simulink model "control_vectorial_bldc"  (R2024b)
settings: Solver=ode14x  StartTime=0.0  StopTime=1  FixedStep=1e-6  MaxStep=1e-5  MinStep=1e-7  RelTol=1e-4  EnableMultiTasking=on
InitFcn:
  | wksp = get_param('control_vectorial_bldc', 'ModelWorkspace');
  | ref_speed = getVariable(wksp, 'w');
  | pw = getVariable(wksp, 'P_speed');
  | iw = getVariable(wksp, 'I_speed');
  | pq = getVariable(wksp, 'P_torque');
  | pd = getVariable(wksp, 'P_flux');
  | pwm_freq = getVariable(wksp, 'pwm_freq');
  | 
  | y = zeros(4, 1000);
  | 
  | command = strcat('sed -i "s/ref_speed =.*/ref_speed = ',num2str(ref_speed),';/" /home/radu/workspace/no-OS/projects/PID_app/src/examples/ext_loop/ext_loop_example.c');
  | [status,cmdout] = system(command);
  | 
  | command = strcat('sed -i "s/pwm_freq =.*/pwm_freq = ',num2str(pwm_freq),';/" /home/radu/workspace/no-OS/projects/PID_app/src/examples/ext_loop/ext_loop_example.c');
  | [status,cmdout] = system(command);
  | 
  | command = strcat('sed -i "s/kp_speed =.*/kp_speed = ',num2str(pw),';/" /home/radu/workspace/no-OS/projects/PID_app/src/examples/ext_loop/ext_loop_example.c');
  | [status,cmdout] = system(command);
  | 
  | command = strcat('sed -i "s/ki_speed =.*/ki_speed = ',num2str(iw),';/" /home/radu/workspace/no-OS/projects/PID_app/src/examples/ext_loop/ext_loop_example.c');
  | [status,cmdout] = system(command);
  | 
  | command = strcat('sed -i "s/kp_torque =.*/kp_torque = ',num2str(pq),';/" /home/radu/workspace/licenta/SOFTWARE/no-OS/projects/PID_app/src/examples/ext_loop/ext_loop_example.c');
  | [status,cmdout] = system(command);
  | 
  | command = strcat('sed -i "s/kp_flux =.*/kp_flux = ',num2str(pd),';/" /home/radu/workspace/no-OS/projects/PID_app/src/examples/ext_loop/ext_loop_example.c');
  | [status,cmdout] = system(command);
  | 
  | cd '/home/radu/workspace/no-OS/projects/PID_app';
  | 
  | command = 'stty -F /dev/ttyACM0 1000000';
  | [status, cmdout] = system(command);
  | command = 'cat /dev/ttyACM0 > speed_plot.txt & make PLATFORM=stm32 run';
  | [status, cmdout] = system(command);
  | 
  | pause(10);
  | 
  | command = 'pkill -f "cat /dev/ttyACM0"';
  | [status, cmdout] = system(command);
  | 
  | fid = fopen('speed_plot.txt','rt');
  | C = textscan(fid, '%f%f%f%f%f%f%f');
  | fclose(fid);
  | y=cell2mat(C);
  | 
  | ms = table2timetable(table(milliseconds(y(:,1:1)), y(:,2:2)));
  | mt = table2timetable(table(milliseconds(y(:,1:1)), y(:,3:3).*0.000009077));
  | mf = table2timetable(table(milliseconds(y(:,1:1)), y(:,4:4).*0.000009077));
  | ms.Properties.VariableNames{1} = 'Motor Speed';
  | mt.Properties.VariableNames{1} = 'Motor Torque';
  | mf.Properties.VariableNames{1} = 'Motor Flux';
  | 
  | command = 'rm speed_plot.txt';
  | [status, cmdout] = system(command);
model workspace (MAT data in the model file):
  I_speed = 0.006
  P_flux = 0.72
  P_speed = 1.04
  P_torque = 0.72
  pwm_freq = 50000
  w = 2000
libraries: ee_lib x15, nesl_utility x10, fl_lib x5, eeTransforms x3, slpidlib x3, spsSVPWMGenerator2LevelLib x1
(part 2 of 2)

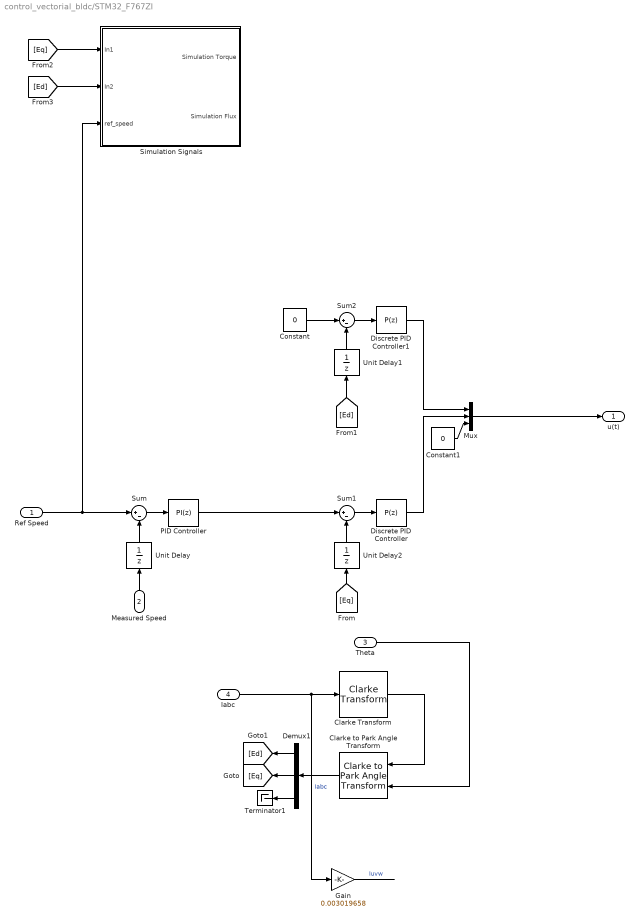
== system control_vectorial_bldc/STM32_F767ZI ==
  Ref Speed : Inport
  Measured Speed : Inport  Port=2
  Theta : Inport  Port=3
  Iabc : Inport  Port=4
  Clarke Transform : eeTransforms/Clarke Transform  PowerInvariant=off
      settings: LibrarySourceBlock=|
      | ee_sl_lib/Mathematical
      | Transforms/Clarke Transform
  Clarke to Park Angle Transform : eeTransforms/Clarke to Park Angle Transform  AxisAlignment=Q-axis
      settings: LibrarySourceBlock=|
      | ee_sl_lib/Mathematical
      | Transforms/Clarke to Park
      | Angle Transform
  Constant : Constant  Value=0
  Constant1 : Constant  Value=0
  Demux1 : Demux  Outputs=3
  Discrete PID Controller : slpidlib/PID Controller  Controller=P  Form=Parallel  TimeDomain=Discrete-time  UseExternalTs=off  SampleTime=-1  IntegratorMethod=Backward Euler  FilterMethod=Forward Euler  ControllerParametersSource=internal  P=P_torque  I=0  UseKiTs=off  D=0  UseExternalDerivativeSource=off  N=100  UseFilter=on  TunerSelectOption=Transfer Function Based (PID Tuner App)  InitialConditionSource=internal  InitialConditionForIntegrator=0  InitialConditionForFilter=0  DifferentiatorICPrevScaledInput=0  ExternalReset=none  TrackingMode=off  Kt=1  LimitOutput=off  SatLimitsSource=internal  UpperSaturationLimit=inf  LowerSaturationLimit=-inf  LinearizeAsGain=off  AntiWindupMode=none  Kb=1  LimitIntegrator=off  UpperIntegratorSaturationLimit=inf  LowerIntegratorSaturationLimit=-inf  POutMin=[]  POutMax=[]  IOutMin=[]  IOutMax=[]  DOutMin=[]  DOutMax=[]  NOutMin=[]  NOutMax=[]  SumOutMin=[]  SumOutMax=[]  SaturationOutMin=[]  SaturationOutMax=[]  PParamMin=[]  PParamMax=[]  IParamMin=[]  IParamMax=[]  DParamMin=[]  DParamMax=[]  NParamMin=[]  NParamMax=[]  KbParamMin=[]  KbParamMax=[]  KtParamMin=[]  KtParamMax=[]  KbOutMin=[]  KbOutMax=[]  KtOutMin=[]  KtOutMax=[]  IntegratorOutMin=[]  IntegratorOutMax=[]  FilterOutMin=[]  FilterOutMax=[]  SumI1OutMin=[]  SumI1OutMax=[]  SumI2OutMin=[]  SumI2OutMax=[]  SumI3OutMin=[]  SumI3OutMax=[]  SumI4OutMin=[]  SumI4OutMax=[]  SumDOutMin=[]  SumDOutMax=[]  DifferentiatorOutMin=[]  DifferentiatorOutMax=[]  FilterDiffOutCoefMin=[]  FilterDiffOutCoefMax=[]  ReciprocalOutMin=[]  ReciprocalOutMax=[]  SumDenOutMin=[]  SumDenOutMax=[]  SumNumOutMin=[]  SumNumOutMax=[]  DivideOutMin=[]  DivideOutMax=[]  UdiffTsProdOutMin=[]  UdiffTsProdOutMax=[]  NTsProdOutMin=[]  NTsProdOutMax=[]  UintegralTsProdOutMin=[]  UintegralTsProdOutMax=[]  UngainTsProdOutMin=[]  UngainTsProdOutMax=[]  ClampingZeroOutDataTypeStr=Inherit: Inherit via back propagation  ClampingZeroOutMin=[]  ClampingZeroOutMax=[]  FilterDenConstantOutDataTypeStr=Inherit: Inherit via back propagation  FilterDenConstantOutMin=[]  FilterDenConstantOutMax=[]  PCopyOutDataTypeStr=Inherit: Inherit via back propagation  PCopyOutMin=[]  PCopyOutMax=[]  NCopyOutDataTypeStr=Inherit: Inherit via back propagation  NCopyOutMin=[]  NCopyOutMax=[]  IntegratorContinuousStateAttributes=''  IntegratorStateMustResolveToSignalObject=off  IntegratorRTWStateStorageClass=Auto  FilterContinuousStateAttributes=''  FilterStateMustResolveToSignalObject=off  FilterRTWStateStorageClass=Auto  ParallelPVariant=InternalParameters  IdealPVariant=Disabled  IVariant=Disabled  DVariant=Disabled  IntegratorVariant=Disabled  SatVariant=Disabled  AWVariant=Disabled  PCopyVariant=Disabled  TRVariant=Disabled  FdbkBlocksVariant=Forward  IdealPFdbkVariant=Disabled  SatFdbkVariant=Disabled  DerivativeFilterVariant=Disabled  NVariant=Disabled  NCopyVariant=Disabled_SignalSpec  FilterICVariant=Disabled  IntegratorICVariant=Disabled  ExternalResetVariant=Disabled  TRSumVariant=Passthrough  SumFdbkVariant=Disabled  SumVariant=Passthrough_P  TsampFilterVariant=InternalTs  TsampNgainVariant=Passthrough  TsampIntegralVariant=Disabled_SignalSpec  ExternalSaturationOutDataTypeStr=Inherit: Same as second input  DerivativeSourceVariant=Disabled  PreIntVariant=InternalPreInt
      settings: LibrarySourceBlock=simulink/Discrete/Discrete PID Controller
  Discrete PID Controller1 : slpidlib/PID Controller  Controller=P  Form=Parallel  TimeDomain=Discrete-time  UseExternalTs=off  SampleTime=-1  IntegratorMethod=Backward Euler  FilterMethod=Forward Euler  ControllerParametersSource=internal  P=P_flux  I=0  UseKiTs=off  D=0  UseExternalDerivativeSource=off  N=100  UseFilter=on  TunerSelectOption=Transfer Function Based (PID Tuner App)  InitialConditionSource=internal  InitialConditionForIntegrator=0  InitialConditionForFilter=0  DifferentiatorICPrevScaledInput=0  ExternalReset=none  TrackingMode=off  Kt=1  LimitOutput=off  SatLimitsSource=internal  UpperSaturationLimit=inf  LowerSaturationLimit=-inf  LinearizeAsGain=off  AntiWindupMode=none  Kb=1  LimitIntegrator=off  UpperIntegratorSaturationLimit=inf  LowerIntegratorSaturationLimit=-inf  POutMin=[]  POutMax=[]  IOutMin=[]  IOutMax=[]  DOutMin=[]  DOutMax=[]  NOutMin=[]  NOutMax=[]  SumOutMin=[]  SumOutMax=[]  SaturationOutMin=[]  SaturationOutMax=[]  PParamMin=[]  PParamMax=[]  IParamMin=[]  IParamMax=[]  DParamMin=[]  DParamMax=[]  NParamMin=[]  NParamMax=[]  KbParamMin=[]  KbParamMax=[]  KtParamMin=[]  KtParamMax=[]  KbOutMin=[]  KbOutMax=[]  KtOutMin=[]  KtOutMax=[]  IntegratorOutMin=[]  IntegratorOutMax=[]  FilterOutMin=[]  FilterOutMax=[]  SumI1OutMin=[]  SumI1OutMax=[]  SumI2OutMin=[]  SumI2OutMax=[]  SumI3OutMin=[]  SumI3OutMax=[]  SumI4OutMin=[]  SumI4OutMax=[]  SumDOutMin=[]  SumDOutMax=[]  DifferentiatorOutMin=[]  DifferentiatorOutMax=[]  FilterDiffOutCoefMin=[]  FilterDiffOutCoefMax=[]  ReciprocalOutMin=[]  ReciprocalOutMax=[]  SumDenOutMin=[]  SumDenOutMax=[]  SumNumOutMin=[]  SumNumOutMax=[]  DivideOutMin=[]  DivideOutMax=[]  UdiffTsProdOutMin=[]  UdiffTsProdOutMax=[]  NTsProdOutMin=[]  NTsProdOutMax=[]  UintegralTsProdOutMin=[]  UintegralTsProdOutMax=[]  UngainTsProdOutMin=[]  UngainTsProdOutMax=[]  ClampingZeroOutDataTypeStr=Inherit: Inherit via back propagation  ClampingZeroOutMin=[]  ClampingZeroOutMax=[]  FilterDenConstantOutDataTypeStr=Inherit: Inherit via back propagation  FilterDenConstantOutMin=[]  FilterDenConstantOutMax=[]  PCopyOutDataTypeStr=Inherit: Inherit via back propagation  PCopyOutMin=[]  PCopyOutMax=[]  NCopyOutDataTypeStr=Inherit: Inherit via back propagation  NCopyOutMin=[]  NCopyOutMax=[]  IntegratorContinuousStateAttributes=''  IntegratorStateMustResolveToSignalObject=off  IntegratorRTWStateStorageClass=Auto  FilterContinuousStateAttributes=''  FilterStateMustResolveToSignalObject=off  FilterRTWStateStorageClass=Auto  ParallelPVariant=InternalParameters  IdealPVariant=Disabled  IVariant=Disabled  DVariant=Disabled  IntegratorVariant=Disabled  SatVariant=Disabled  AWVariant=Disabled  PCopyVariant=Disabled  TRVariant=Disabled  FdbkBlocksVariant=Forward  IdealPFdbkVariant=Disabled  SatFdbkVariant=Disabled  DerivativeFilterVariant=Disabled  NVariant=Disabled  NCopyVariant=Disabled_SignalSpec  FilterICVariant=Disabled  IntegratorICVariant=Disabled  ExternalResetVariant=Disabled  TRSumVariant=Passthrough  SumFdbkVariant=Disabled  SumVariant=Passthrough_P  TsampFilterVariant=InternalTs  TsampNgainVariant=Passthrough  TsampIntegralVariant=Disabled_SignalSpec  ExternalSaturationOutDataTypeStr=Inherit: Same as second input  DerivativeSourceVariant=Disabled  PreIntVariant=InternalPreInt
      settings: LibrarySourceBlock=simulink/Discrete/Discrete PID Controller
  Gain : Gain  Gain=0.003019658
  Mux : Mux  Inputs=3
  PID Controller : slpidlib/PID Controller  Controller=PI  Form=Parallel  TimeDomain=Discrete-time  UseExternalTs=off  SampleTime=5e-4  IntegratorMethod=Backward Euler  FilterMethod=Forward Euler  ControllerParametersSource=internal  P=P_speed  I=I_speed  UseKiTs=off  D=1  UseExternalDerivativeSource=off  N=100  UseFilter=on  TunerSelectOption=Transfer Function Based (PID Tuner App)  InitialConditionSource=internal  InitialConditionForIntegrator=0  InitialConditionForFilter=0  DifferentiatorICPrevScaledInput=0  ExternalReset=none  TrackingMode=off  Kt=1  LimitOutput=off  SatLimitsSource=internal  UpperSaturationLimit=inf  LowerSaturationLimit=-inf  LinearizeAsGain=on  AntiWindupMode=none  Kb=1  LimitIntegrator=off  UpperIntegratorSaturationLimit=inf  LowerIntegratorSaturationLimit=-inf  POutMin=[]  POutMax=[]  IOutMin=[]  IOutMax=[]  DOutMin=[]  DOutMax=[]  NOutMin=[]  NOutMax=[]  SumOutMin=[]  SumOutMax=[]  SaturationOutMin=[]  SaturationOutMax=[]  PParamMin=[]  PParamMax=[]  IParamMin=[]  IParamMax=[]  DParamMin=[]  DParamMax=[]  NParamMin=[]  NParamMax=[]  KbParamMin=[]  KbParamMax=[]  KtParamMin=[]  KtParamMax=[]  KbOutMin=[]  KbOutMax=[]  KtOutMin=[]  KtOutMax=[]  IntegratorOutMin=[]  IntegratorOutMax=[]  FilterOutMin=[]  FilterOutMax=[]  SumI1OutMin=[]  SumI1OutMax=[]  SumI2OutMin=[]  SumI2OutMax=[]  SumI3OutMin=[]  SumI3OutMax=[]  SumI4OutMin=[]  SumI4OutMax=[]  SumDOutMin=[]  SumDOutMax=[]  DifferentiatorOutMin=[]  DifferentiatorOutMax=[]  FilterDiffOutCoefMin=[]  FilterDiffOutCoefMax=[]  ReciprocalOutMin=[]  ReciprocalOutMax=[]  SumDenOutMin=[]  SumDenOutMax=[]  SumNumOutMin=[]  SumNumOutMax=[]  DivideOutMin=[]  DivideOutMax=[]  UdiffTsProdOutMin=[]  UdiffTsProdOutMax=[]  NTsProdOutMin=[]  NTsProdOutMax=[]  UintegralTsProdOutMin=[]  UintegralTsProdOutMax=[]  UngainTsProdOutMin=[]  UngainTsProdOutMax=[]  ClampingZeroOutDataTypeStr=Inherit: Inherit via back propagation  ClampingZeroOutMin=[]  ClampingZeroOutMax=[]  FilterDenConstantOutDataTypeStr=Inherit: Inherit via back propagation  FilterDenConstantOutMin=[]  FilterDenConstantOutMax=[]  PCopyOutDataTypeStr=Inherit: Inherit via back propagation  PCopyOutMin=[]  PCopyOutMax=[]  NCopyOutDataTypeStr=Inherit: Inherit via back propagation  NCopyOutMin=[]  NCopyOutMax=[]  IntegratorContinuousStateAttributes=''  IntegratorStateMustResolveToSignalObject=off  IntegratorRTWStateStorageClass=Auto  FilterContinuousStateAttributes=''  FilterStateMustResolveToSignalObject=off  FilterRTWStateStorageClass=Auto  ParallelPVariant=InternalParameters  IdealPVariant=Disabled  IVariant=InternalParameters  DVariant=Disabled  IntegratorVariant=Discrete  SatVariant=Disabled  AWVariant=Passthrough  PCopyVariant=Disabled  TRVariant=Disabled  FdbkBlocksVariant=Forward  IdealPFdbkVariant=Disabled  SatFdbkVariant=Disabled  DerivativeFilterVariant=Disabled  NVariant=Disabled  NCopyVariant=Disabled_SignalSpec  FilterICVariant=Disabled  IntegratorICVariant=InternalICs  ExternalResetVariant=Disabled  TRSumVariant=Passthrough  SumFdbkVariant=Disabled  SumVariant=Sum_PI  TsampFilterVariant=InternalTs  TsampNgainVariant=Passthrough  TsampIntegralVariant=Disabled_SignalSpec  ExternalSaturationOutDataTypeStr=Inherit: Same as second input  DerivativeSourceVariant=Disabled  PreIntVariant=InternalPreInt
  Simulation Signals : Subsystem
  Sum : Sum  Inputs=|+-
  Sum1 : Sum  Inputs=|+-
  Sum2 : Sum  Inputs=|+-
  Terminator1 : Terminator
  Unit Delay : UnitDelay  SampleTime=1e-5  HasFrameUpgradeWarning=on
  Unit Delay1 : UnitDelay  SampleTime=1e-5  HasFrameUpgradeWarning=on
  Unit Delay2 : UnitDelay  SampleTime=1e-5  HasFrameUpgradeWarning=on
  u(t) : Outport
  wires:
  Sum/1 -> PID Controller/1
  Ref Speed/1 -> Simulation Signals/3(ref_speed), Sum/1
  Sum1/1 -> Discrete PID Controller/1
  Sum2/1 -> Discrete PID Controller1/1
  Constant1/1 -> Mux/3
  Clarke to Park Angle Transform/1 -> Demux1/1
  Demux1/3 -> Terminator1/1
  Unit Delay/1 -> Sum/2
  Unit Delay1/1 -> Sum2/2
  Unit Delay2/1 -> Sum1/2
  Discrete PID Controller1/1 -> Mux/1
  Discrete PID Controller/1 -> Mux/2
  Measured Speed/1 -> Unit Delay/1
  Theta/1 -> Clarke to Park Angle Transform/2
  Iabc/1 -> Clarke Transform/1, Gain/1  "Iabc"
  Demux1/2 -> [Eq]
  [Eq] -> Unit Delay2/1
  [Ed] -> Unit Delay1/1
  Demux1/1 -> [Ed]
  Constant/1 -> Sum2/1
  Clarke Transform/1 -> Clarke to Park Angle Transform/1
  Mux/1 -> u(t)/1
  PID Controller/1 -> Sum1/1
  [Eq] -> Simulation Signals/1(In1)
  [Ed] -> Simulation Signals/2(In2)
  Gain/1 -> ?  "Iuvw"

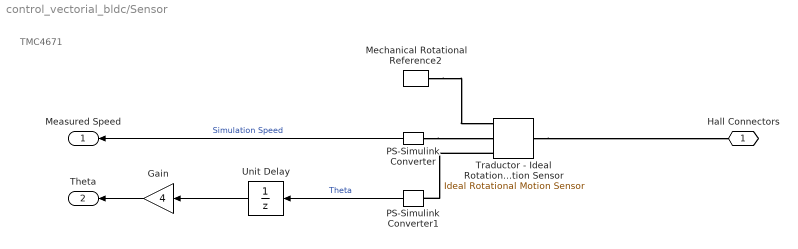
== system control_vectorial_bldc/Sensor ==
  note: TMC4671
  Gain : Gain  Gain=4
  Mechanical Rotational Reference2 : fl_lib/Mechanical/Rotational Elements/Mechanical Rotational Reference
  PS-Simulink Converter : nesl_utility/PS-Simulink Converter  PhysicalDomain=network_engine_domain  SubClassName=ps_output  LeftPortType=input  RightPortType=output  PseudoPeriodic=off  Frequencies=[]  VectorFormat=inherit  Unit=rpm  AffineConversion=off
  PS-Simulink Converter1 : nesl_utility/PS-Simulink Converter  PhysicalDomain=network_engine_domain  SubClassName=ps_output  LeftPortType=input  RightPortType=output  PseudoPeriodic=off  Frequencies=[]  VectorFormat=inherit  Unit=rad  AffineConversion=off
  Traductor - Ideal Rotational Motion Sensor : fl_lib/Mechanical/Mechanical Sensors/Ideal Rotational Motion Sensor  reference=foundation.enum.MeasurementReference.difference  acceleration_port=false  velocity_port=true  position_port=true  wrap_angle=false  offset=0 deg
  Unit Delay : UnitDelay  SampleTime=-1  HasFrameUpgradeWarning=on
  Hall Connectors : PMIOPort  Side=Left
  Measured Speed : Outport
  Theta : Outport  Port=2
  wires:
  PS-Simulink Converter1/1 -> Unit Delay/1  "Theta"
  Gain/1 -> Theta/1
  PS-Simulink Converter/1 -> Measured Speed/1  "Simulation Speed"
  Unit Delay/1 -> Gain/1
  connections:
  PS-Simulink Converter/LConn1 -- Traductor - Ideal Rotational Motion Sensor/RConn2
  Traductor - Ideal Rotational Motion Sensor/RConn3 -- PS-Simulink Converter1/LConn1
  Mechanical Rotational Reference2/LConn1 -- Traductor - Ideal Rotational Motion Sensor/RConn1
  Traductor - Ideal Rotational Motion Sensor/LConn1 -- Hall Connectors/RConn1

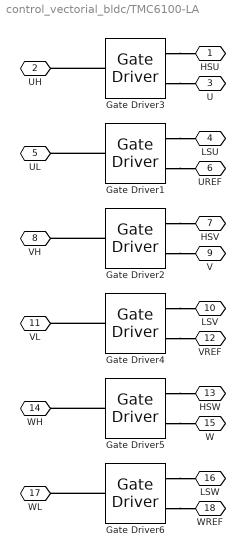
== system control_vectorial_bldc/TMC6100-LA ==
  Gate Driver{1..6} (6 alike) : ee_lib/Semiconductors & Converters/Gate Driver  port_option=ee.enum.controlport.ps  uHigh=3.3 V  uLow=0 V  uHighValue=2.31  uLowValue=0.99  vHigh=12 V  vLow=0 V  tHigh=85 ns  tLow=85 ns  parameterization=ee.enum.semiconductors.gateDriverParam.riseAndFallTimes  rHigh=2 Ohm  rLow=1.3 Ohm  tRise=10 ns  tFall=10 ns  cLoad=10 nF  t_fault=1 s  ZonTime_specify=off  ZonTime_priority=None  ZonTime=0 s  ZoffTime_specify=off  ZoffTime_priority=None  ZoffTime=0 s
      settings: InternalSimscapePortConfiguration="{\"Bottom\":[],\"Left\":[{\"id\":\"u\",\"label\":\"u\",\"type\":\"input\"}],\"Right\":[{\"id\":\"G\",\"label\":\"G\",\"type\":\"foundation.electrical.electrical\"},{\"id\":\"S\",\"label\":\"S\",\"type\":\"foundation.electrical.electrical\"}],\"Top\":[]}"
  HSU : PMIOPort  Side=Right
  UH : PMIOPort  Port=2  Side=Left
  U : PMIOPort  Port=3  Side=Right
  LSU : PMIOPort  Port=4  Side=Right
  UL : PMIOPort  Port=5  Side=Left
  UREF : PMIOPort  Port=6  Side=Right
  HSV : PMIOPort  Port=7  Side=Right
  VH : PMIOPort  Port=8  Side=Left
  V : PMIOPort  Port=9  Side=Right
  "LSV " : PMIOPort  Port=10  Side=Right
  VL : PMIOPort  Port=11  Side=Left
  VREF : PMIOPort  Port=12  Side=Right
  HSW : PMIOPort  Port=13  Side=Right
  WH : PMIOPort  Port=14  Side=Left
  W : PMIOPort  Port=15  Side=Right
  LSW : PMIOPort  Port=16  Side=Right
  WL : PMIOPort  Port=17  Side=Left
  WREF : PMIOPort  Port=18  Side=Right
  connections:
  Gate Driver1/RConn2 -- UREF/RConn1
  Gate Driver3/RConn2 -- U/RConn1
  Gate Driver5/RConn2 -- W/RConn1
  Gate Driver4/RConn2 -- VREF/RConn1
  Gate Driver3/RConn1 -- HSU/RConn1
  Gate Driver5/RConn1 -- HSW/RConn1
  Gate Driver2/RConn2 -- V/RConn1
  Gate Driver2/RConn1 -- HSV/RConn1
  Gate Driver4/RConn1 -- "LSV "/RConn1
  Gate Driver6/RConn1 -- LSW/RConn1
  Gate Driver1/RConn1 -- LSU/RConn1
  Gate Driver6/RConn2 -- WREF/RConn1
  Gate Driver3/LConn1 -- UH/RConn1
  Gate Driver1/LConn1 -- UL/RConn1
  Gate Driver2/LConn1 -- VH/RConn1
  Gate Driver4/LConn1 -- VL/RConn1
  Gate Driver5/LConn1 -- WH/RConn1
  Gate Driver6/LConn1 -- WL/RConn1

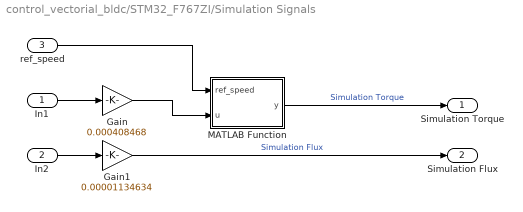
== system control_vectorial_bldc/STM32_F767ZI/Simulation Signals ==
  In1 : Inport
  In2 : Inport  Port=2
  ref_speed : Inport  Port=3
  Gain : Gain  Gain=0.000408468
  Gain1 : Gain  Gain=0.00001134634
  MATLAB Function : MATLAB Function  TreatAsAtomicUnit=on
  Simulation Torque : Outport
  Simulation Flux : Outport  Port=2
  wires:
  In2/1 -> Gain1/1
  Gain1/1 -> Simulation Flux/1  "Simulation Flux"
  In1/1 -> Gain/1
  Gain/1 -> MATLAB Function/2(u)
  MATLAB Function/1(y) -> Simulation Torque/1  "Simulation Torque"
  ref_speed/1 -> MATLAB Function/1(ref_speed)

== matlab function control_vectorial_bldc/STM32_F767ZI/Simulation Signals/MATLAB Function ==
  data: ref_speed input; u input; y output
function y = fcn(ref_speed, u)

if (ref_speed < 0 && u > 0)
    u = 0;
end

if (ref_speed > 0 && u < 0)
    u = 0;
end

y = u;
